simulink model "While_Loop_in_Stateflow"  (R2018b)
settings: Solver=FixedStepDiscrete  StartTime=0.0  StopTime=10.0  RelTol=1e-3
libraries: simulink x1
settings Model: Creator=marwan  LastModifiedBy=marwan

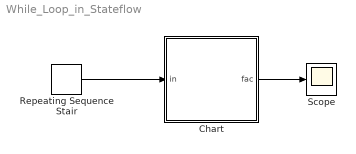
== system While_Loop_in_Stateflow ==
  Chart : Stateflow chart  TreatAsAtomicUnit=on
  Repeating Sequence Stair : simulink/Sources/Repeating Sequence Stair  OutValues=[1 2 3 4 5].'  tsamp=-1  OutMin=[]  OutMax=[]  OutDataTypeStr=double  OutputDataTypeScalingMode=double  OutDataType=fixdt(0,8)  ConRadixGroup=Best Precision: Vector-wise  OutScaling=2^-12
  Scope : Scope
  wires:
  Chart/1(fac) -> Scope/1
  Repeating Sequence Stair/1 -> Chart/1(in)

== stateflow chart While_Loop_in_Stateflow/Chart ==
  (default) -> (junction 9)
  (junction 11) -> (junction 10) [order 1] : [temp>=1]
  (junction 9) -> (junction 11) : {mul=1;
      | temp=in;}
  (junction 10) -> (junction 12) : {mul=mul*temp;
      | temp=temp-1;}
  (junction 12) -> (junction 11)
  (junction 11) -> (junction 13) [order 2] : {fac=mul;}
  data: in input; fac output; mul local; temp local
